simulink model "Test_GenericClient"  (R2019a)
settings: Solver=FixedStepDiscrete  StartTime=0.0  StopTime=10  RelTol=1e-6  AbsTol=1e-6  EnableMultiTasking=on
InitFcn:
  | clear('all');
libraries: simulink x1
settings Model: Creator=Andreas Schellenberg  LastModifiedBy=Andreas
settings SolverCC: AutoScaleAbsTol=off
settings DataIOCC: SaveFormat=StructureWithTime  SignalLoggingSaveFormat=ModelDataLogs  SaveState=on  SignalLogging=off  ReturnWorkspaceOutputs=off  SignalLoggingName=sigsOut  OutputOption=SpecifiedOutputTimes  OutputTimes=t
settings OptimizationCC: ExpressionDepthLimit=2147483647  InitFltsAndDblsToZero=on  LifeSpan=inf
settings DebuggingCC: SaveWithParameterizedLinksMsg=none  UnderspecifiedInitializationDetection=Classic  MergeDetectMultiDrivingBlocksExec=none  SignalResolutionControl=TryResolveAllWithWarning  MultiTaskDSMMsg=warning  MultiTaskCondExecSysMsg=none  FcnCallInpInsideContextMsg=warning  StateNameClashWarn=warning  SFUnexpectedBacktrackingDiag=warning  SFNoUnconditionalDefaultTransitionDiag=warning  SFExecutionAtInitializationDiag=none  ArithmeticOperatorsInVariantConditions=warning
settings HardwareCC: ProdBitPerPointer=32  ProdBitPerSizeT=32  ProdBitPerPtrDiffT=32  ProdLargestAtomicFloat=None  ProdIntDivRoundTo=Undefined  ProdEndianess=Unspecified  ProdWordSize=32  ProdHWDeviceType=32-bit Generic  TargetUnknown=on
settings ModelReferenceCC: PropagateSignalLabelsOutOfModel=off
settings SFSimCC: SimUseLocalCustomCode=off
settings RTWCC: RTWUseLocalCustomCode=off
settings CodeAppCC: StateflowObjectComments=on
settings GRTTargetCC: TargetLangStandard=C89/C90 (ANSI)  CombineOutputUpdateFcns=off  GRTInterface=on
settings ConfigComp: CovMetricSettings=dw  CovHtmlReporting=on  CovSaveCumulativeToWorkspaceVar=on  CovSaveSingleToWorkspaceVar=on

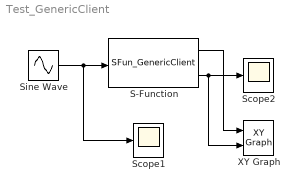
== system Test_GenericClient ==
  S-Function : S-Function  FunctionName=SFun_GenericClient  Parameters=ipAddr,ipPort,dataSize  SFunctionDeploymentMode=off  EnableBusSupport=off  mask(GenericClient Element){ipAddr=127.0.0.1, ipPort=8090, dataSize=256}
      mask prompts: ipAddr "IP Address of Server"; ipPort "IP Port Number of Server"; dataSize "Size of Data Arrays"
      mask Display: disp('GenericClient\nElement');
  Scope1 : Scope
  Scope2 : Scope
  Sine Wave : Sin  Amplitude=2  Frequency=pi  SampleTime=0.01
  XY Graph : simulink/Sinks/XY Graph  xmin=-2.5  xmax=2.5  ymin=-2  ymax=2  st=-1
  wires:
  Sine Wave/1 -> S-Function/1, Scope1/1
  S-Function/2 -> Scope2/1, XY Graph/2
  S-Function/1 -> XY Graph/1
